simulink model "Greedy_Delay_u"  (R2015a)
settings: Solver=ode3  StartTime=0.0  StopTime=350  FixedStep=0.01  MaxStep=0.01  RelTol=1e-3
values from neighbouring files (symbols this model uses):
  H0 = interp1q(Periodic_Solution(:,1),Periodic_Solution(:,4),time_shift(n))    [Gradient_Descent_Controllable_Sleeping.m]
  Periodic_Solution = Periodic_Solution(Initial_Time*100+1:end,:)    [Gradient_Descent_Controllable_Sleeping.m]    (also in Periodic_Solution_JFK_u_1000lux.mat = [0 0.00999999999999 0.02 0.03 0.04 0.05 0.0599999999999 0.06)
  tol = 0.01    [Gradient_Descent_Controllable_Sleeping.m]
  umax = 0.2208    [Gradient_Descent_Controllable_Sleeping.m]
  x0 = interp1q(Periodic_Solution(:,1),Periodic_Solution(:,2),time_shift(n))    [Gradient_Descent_Controllable_Sleeping.m]
  xc0 = interp1q(Periodic_Solution(:,1),Periodic_Solution(:,3),time_shift(n))    [Gradient_Descent_Controllable_Sleeping.m]
undefined symbols (not defined in the file or in its folder): f
settings Model: Creator=wangf7  LastModifiedBy=Jiawei Yin
settings OptimizationCC: ExpressionDepthLimit=2147483647
settings DebuggingCC: AlgebraicLoopMsg=none  ArtificialAlgebraicLoopMsg=none  UnderspecifiedInitializationDetection=Classic  MergeDetectMultiDrivingBlocksExec=none  SolverPrmCheckMsg=warning  StateNameClashWarn=warning

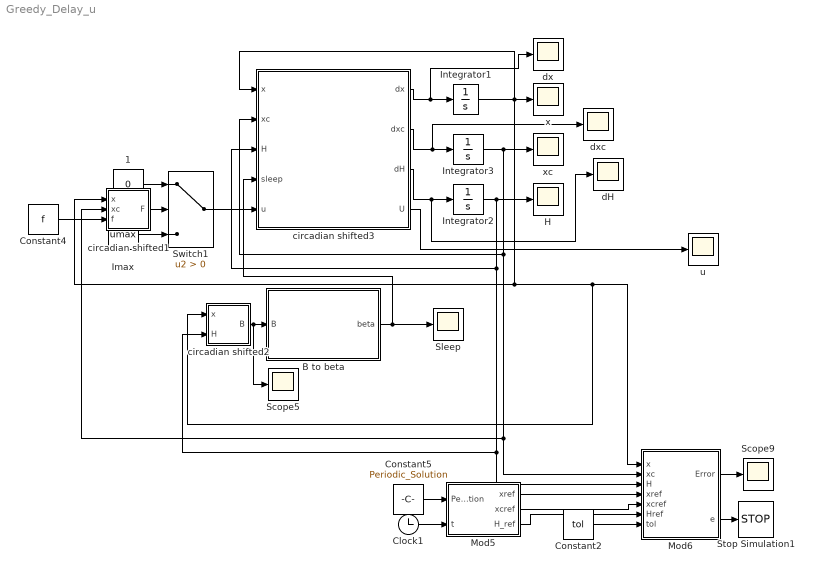
== system Greedy_Delay_u ==
  1 : Constant  Value=0
  "B to beta " : Subsystem
  Clock1 : Clock
  Constant2 : Constant  Value=tol
  Constant4 : Constant  Value=f
  Constant5 : Constant  Value=Periodic_Solution
  H : Scope
      settings: TimeRange=auto  MaxDataPoints=5000000000  SaveName=H  YMin=0.0513  YMax=0.6724  SampleTime=-1  DataFormat=Array
  Imax : Constant  Value=umax
  Integrator1 : Integrator  InitialCondition=x0
  Integrator2 : Integrator  InitialCondition=H0
  Integrator3 : Integrator  InitialCondition=xc0
  Mod5 : MATLAB Function  TreatAsAtomicUnit=on
      settings: PermitHierarchicalResolution=ParametersOnly
  Mod6 : MATLAB Function  TreatAsAtomicUnit=on
      settings: PermitHierarchicalResolution=ParametersOnly
  Scope5 : Scope
      settings: TimeRange=auto  MaxDataPoints=5000000000  SaveName=B  YMin=0.02521  YMax=0.68144  SampleTime=-1  DataFormat=Array
  Scope9 : Scope
      settings: TimeRange=auto  LimitDataPoints=on  MaxDataPoints=5000000000  SaveName=Error  YMin=0.03979635839198  YMax=0.03979635839227  SampleTime=-1  DataFormat=Array
  Sleep : Scope
      settings: TimeRange=auto  MaxDataPoints=5000000000  SaveName=Sleep  YMin=-0.125  YMax=1.125  SampleTime=-1  DataFormat=Array
  Stop Simulation1 : Stop
  Switch1 : Switch  Criteria=u2 > Threshold
  circadian shifted1 : MATLAB Function  TreatAsAtomicUnit=on
      settings: PermitHierarchicalResolution=ParametersOnly
  circadian shifted2 : MATLAB Function  TreatAsAtomicUnit=on
      settings: PermitHierarchicalResolution=ParametersOnly
  circadian shifted3 : MATLAB Function  TreatAsAtomicUnit=on
      settings: PermitHierarchicalResolution=ParametersOnly
  dH : Scope
      settings: TimeRange=auto  MaxDataPoints=5000000000  SaveName=dH  YMin=0.0513  YMax=0.6724  SampleTime=-1  DataFormat=Array
  dx : Scope
      settings: TimeRange=auto  MaxDataPoints=5000000000  SaveName=dx  YMin=-0.69121  YMax=1.2048  SampleTime=-1  DataFormat=Array
  dxc : Scope
      settings: TimeRange=auto  MaxDataPoints=5000000000  SaveName=dxc  YMin=-1.51575  YMax=1.31005  SampleTime=-1  DataFormat=Array
  u : Scope
      settings: TimeRange=auto  MaxDataPoints=5000000000  SaveName=u  YMin=-0.125  YMax=1.125  SampleTime=-1  DataFormat=Array
  x : Scope
      settings: TimeRange=auto  MaxDataPoints=5000000000  SaveName=x  YMin=-0.69121  YMax=1.2048  SampleTime=-1  DataFormat=Array
  xc : Scope
      settings: TimeRange=auto  MaxDataPoints=5000000000  SaveName=xc  YMin=-1.51575  YMax=1.31005  SampleTime=-1  DataFormat=Array
  wires:
  Imax/1 -> Switch1/3
  Constant4/1 -> circadian shifted1/3(f)
  circadian shifted3/1(dx) -> dx/1, Integrator1/1
  circadian shifted3/2(dxc) -> dxc/1, Integrator3/1
  Integrator1/1 -> Mod6/1(x), circadian shifted2/1(x), circadian shifted1/1(x), circadian shifted3/1(x), x/1
  Integrator3/1 -> Mod6/2(xc), circadian shifted1/2(xc), circadian shifted3/2(xc), xc/1
  circadian shifted2/1(B) -> Scope5/1, "B to beta "/1(B)
  "B to beta "/1(beta) -> circadian shifted3/4(sleep), Sleep/1
  Constant5/1 -> Mod5/1(Periodic_Solution)
  Clock1/1 -> Mod5/2(t)
  Mod6/2(e) -> Stop Simulation1/1
  Mod6/1(Error) -> Scope9/1
  circadian shifted1/1(F) -> Switch1/2
  Constant2/1 -> Mod6/7(tol)
  circadian shifted3/3(dH) -> dH/1, Integrator2/1
  Integrator2/1 -> H/1, circadian shifted2/2(H), Mod6/3(H), circadian shifted3/3(H)
  Switch1/1 -> circadian shifted3/5(u)
  Mod5/1(xref) -> Mod6/4(xref)
  Mod5/2(xcref) -> Mod6/5(xcref)
  Mod5/3(H_ref) -> Mod6/6(Href)
  1/1 -> Switch1/1
  circadian shifted3/4(U) -> u/1

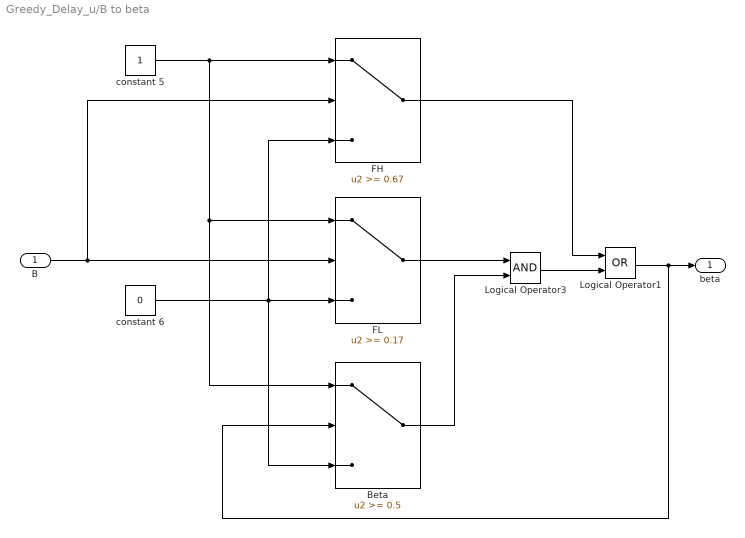
== system Greedy_Delay_u/B to beta  ==
  B : Inport
  Beta : Switch  Threshold=0.5
  FH : Switch  Threshold=0.67
  FL : Switch  Threshold=0.17
  Logical Operator1 : Logic  Operator=OR  AllPortsSameDT=off  OutDataTypeStr=boolean
  Logical Operator3 : Logic  AllPortsSameDT=off  OutDataTypeStr=boolean
  constant 5 : Constant
  constant 6 : Constant  Value=0
  beta : Outport
  wires:
  constant 5/1 -> Beta/1, FL/1, FH/1
  constant 6/1 -> Beta/3, FH/3, FL/3
  B/1 -> FH/2, FL/2
  Logical Operator1/1 -> Beta/2, beta/1
  FL/1 -> Logical Operator3/1
  Beta/1 -> Logical Operator3/2
  Logical Operator3/1 -> Logical Operator1/2
  FH/1 -> Logical Operator1/1

== matlab function Greedy_Delay_u/circadian shifted1 ==
  data: x input; xc input; f input; F output
function F = fcn(x,xc,f)
%#eml
F=interp1q(f(:,1),f(:,2),mod(atan2(-xc,x),2*pi));

== matlab function Greedy_Delay_u/circadian shifted3 ==
  data: x input; xc input; H input; sleep input; u input; dx output; dxc output; dH output; U output
function [ dx,dxc,dH,U] = fcn(x,xc,H,sleep,u)
%#eml

tr=18.2;
td=4.2;

q = 1/3;
taux = 24.2;
k = 0.55;
mu=0.13;
U=u*(1-sleep);
B = u*(1-0.4*x)*(1-0.4*xc)*(1-sleep);

dx = (pi/12)*(xc + B  + mu*(1/3*x + 4/3*x^3 - 256/105*x^7));
dxc = (pi/12)*(q*B *xc - (24/(taux*0.99729))^2*x - k*B*x);
dH = (1-sleep)*(1-H)/tr-(H*sleep)/td;

== matlab function Greedy_Delay_u/circadian shifted2 ==
  data: x input; H input; B output
function B = fcn(x,H)
%#eml
B=H-0.1333*x;

== matlab function Greedy_Delay_u/Mod5 ==
  data: Periodic_Solution input; xref output; xcref output; t input; H_ref output
function [xref,xcref,H_ref] = fcn(Periodic_Solution,t)
%#codegen
xref=interp1q(Periodic_Solution(:,1),Periodic_Solution(:,2),t);
xcref=interp1q(Periodic_Solution(:,1),Periodic_Solution(:,3),t);
H_ref=interp1q(Periodic_Solution(:,1),Periodic_Solution(:,4),t);
% sleep_ref=interp1q(Periodic_Solution(:,1),Periodic_Solution(:,6),t);

== matlab function Greedy_Delay_u/Mod6 ==
  data: Error output; x input; xc input; H input; e output; xref input; xcref input; Href input; tol input
function [Error,e] = fcn(x,xc,H,xref,xcref,Href,tol)
%#codegen
Error=(H-Href)^2+(x-xref)^2+(xc-xcref)^2;
e=Error<tol;
